simulink model "practice"  (R2024b)
settings: Solver=VariableStepAuto  StartTime=0.0  StopTime=15.0  RelTol=1e-3
settings Model: Creator=andrey  LastModifiedBy=andrey

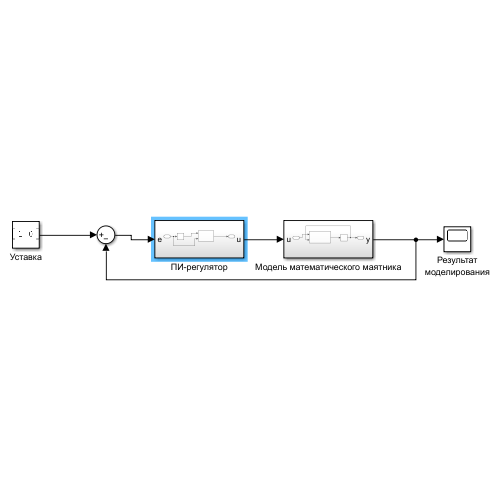
[thumbnail: Simulink's stored preview of the top-level diagram]
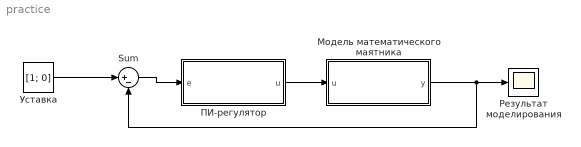
== system practice ==
  Sum : Sum  Inputs=|+-
  Модель математического маятника : Subsystem
  ПИ-регулятор : Subsystem
  Результат моделирования : Scope
  Уставка : Constant  Value=[1; 0]
  wires:
  Уставка/1 -> Sum/1
  Sum/1 -> ПИ-регулятор/1(e)
  ПИ-регулятор/1(u) -> Модель математического маятника/1(u)
  Модель математического маятника/1(y) -> Результат моделирования/1, Sum/2

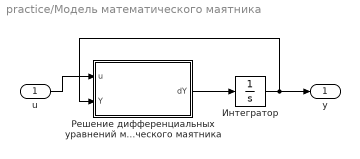
== system practice/Модель математического маятника ==
  u : Inport
  Интегратор : Integrator  InitialCondition=[-2; 0]
  Решение дифференциальных уравнений математического маятника : MATLAB Function  TreatAsAtomicUnit=on
  y : Outport
  wires:
  Решение дифференциальных уравнений математического маятника/1(dY) -> Интегратор/1
  Интегратор/1 -> Решение дифференциальных уравнений математического маятника/2(Y), y/1
  u/1 -> Решение дифференциальных уравнений математического маятника/1(u)

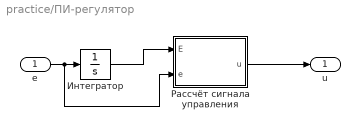
== system practice/ПИ-регулятор ==
  e : Inport
  Интегратор : Integrator  InitialCondition=[-2;0]
  Рассчёт сигнала управления : MATLAB Function  TreatAsAtomicUnit=on
  u : Outport
  wires:
  Рассчёт сигнала управления/1(u) -> u/1
  Интегратор/1 -> Рассчёт сигнала управления/1(E)
  e/1 -> Рассчёт сигнала управления/2(e), Интегратор/1

== matlab function practice/Модель математического маятника/Решение дифференциальных уравнений математического маятника ==
  data: u input; Y input; dY output
function dY = koshi(u, Y)
g = 9.81;
l = 0.1;
m= 0.5;
b = 1;
c = 1;

dY = zeros(length(Y), 1);
dY(1) = Y(2);
dY(2) = -g/l * sin(Y(1)) - b/(m*l*l) * dY(1) - c/(m*l*l) * Y(1) - u/(m*l*l);
end

== matlab function practice/ПИ-регулятор/Рассчёт сигнала управления ==
  data: E input; u output; e input
function u = control(E, e)
Kp = 0.654;
Ki = -0.654;
u = Kp * e(1) + Kp * e(2) + Ki * E(1) + Ki * E(2);
end
